simulink model "week8_trial"  (R2020b)
settings: Solver=VariableStepAuto  StartTime=0.0  StopTime=100  FixedStep=0.1  RelTol=1e-3
undefined symbols (not defined in the file or in its folder): Cf, Cr, Iz, lf, lr, m, md, sigbuilder_block, Ts, V_init
libraries: pid_lib x2, mpcadaslib x1
(part 1 of 2)
settings Model: Creator=anime  LastModifiedBy=anime

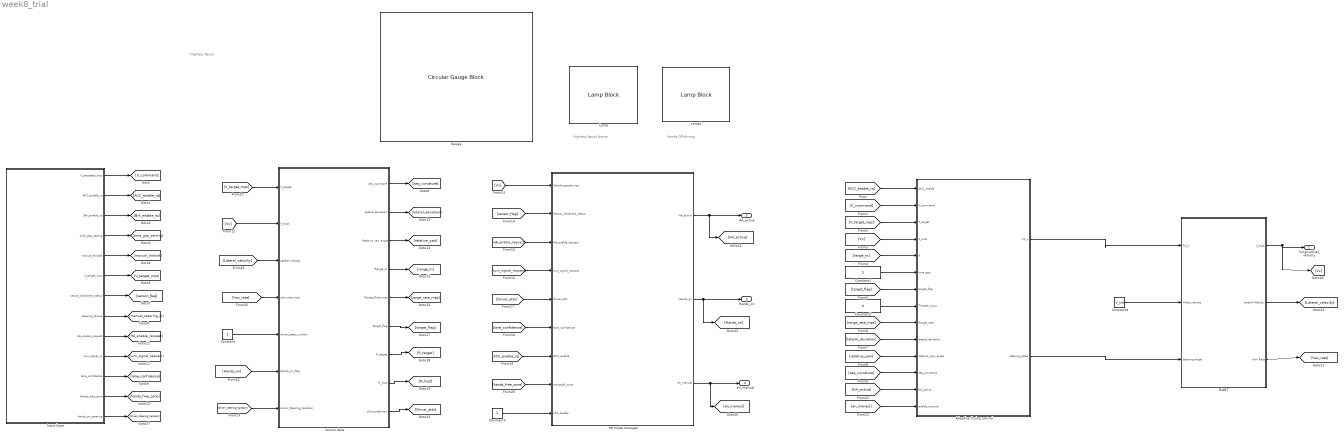
== system week8_trial ==
  note: Hands Off driving
  note: Highway Assist
  note: Highway Assist Active
  Adaptive Cruise control : Subsystem
  Constant : Constant
  Constant1 : Constant  Value=3
  Constant2 : Constant  Value=0
  Constant3 : Constant
  Constant4 : Constant  Value=V_init
  Gauge : CircularGaugeBlock  LabelPosition=Bottom  ScaleMax=50
  HA mode manager : Subsystem
  Input layer : Subsystem
  Lamp : LampBlock  LabelPosition=Bottom
  Lamp1 : LampBlock  LabelPosition=Bottom
  PLANT : Subsystem
  "Sensor data " : Subsystem
  longitudinal_velocity : Outport  Unit=m/s  VectorParamsAs1DForOutWhenUnconnected=off
  HA_active : Outport  Port=2
  Hands_on : Outport  Port=3
  en_manual : Outport  Port=4
  wires:
  Input layer/5(manual_throttle) -> [manual_throttle]
  Input layer/12(Hands_free_zone) -> [hands_free_zone]
  Input layer/11(lane_confidence) -> [lane_confidence]
  Input layer/10(turn_signal_rq) -> [turn_signal_request]
  Input layer/6(V_target_mps) -> [V_target_mps]
  Input layer/9(HA_enable_request) -> [HA_enable_request]
  Input layer/3(Brk_enable_rq) -> [Brk_enable_rq]
  Input layer/8(steering_torque) -> [manual_steering_io]
  Input layer/7(sensor_hardware_status) -> [sensor_flag]
  Input layer/4(time_gap_setting) -> [time_gap_setting]
  Input layer/1(V_setspeed_mps) -> [V_command]
  Input layer/2(ACC_enable_rq) -> [ACC_enable_rq]
  "Sensor data "/9(drive_attention) -> [Driver_attn]
  "Sensor data "/6(Target_flag) -> [target_flag]
  [Yaw_rate] -> "Sensor data "/4(yaw_rate_mps)
  "Sensor data "/8(R_host) -> [R_host]
  "Sensor data "/7(R_target) -> [R_target]
  "Sensor data "/4(Range_m) -> [range_m]
  "Sensor data "/3(Relative yaw angle) -> [relative_yaw]
  [Vx] -> "Sensor data "/2(V_host)
  "Sensor data "/5(Range_Rate_mps) -> [range_rate_mps]
  "Sensor data "/2(Lateral deviation) -> [lateral_deviation]
  [V_target_mps] -> "Sensor data "/1(V_target)
  [Lateral_velocity] -> "Sensor data "/3(Lateral velocity)
  Constant/1 -> "Sensor data "/5(driver_state_monitor)
  "Sensor data "/1(seq_curvature) -> [seq_curvature]
  Constant4/1 -> PLANT/2(initial_velocity)
  [ACC_enable_rq] -> Adaptive Cruise control/1(ACC_enable)
  [V_command] -> Adaptive Cruise control/2(V_command)
  [V_target_mps] -> Adaptive Cruise control/3(V_target)
  [Vx] -> Adaptive Cruise control/4(V_host)
  [range_m] -> Adaptive Cruise control/5(R)
  [target_flag] -> Adaptive Cruise control/7(target_flag)
  Constant1/1 -> Adaptive Cruise control/6(time gap)
  Constant2/1 -> Adaptive Cruise control/8(Throttle_input)
  [range_rate_mps] -> Adaptive Cruise control/9(Range_rate)
  Adaptive Cruise control/1(Fd_u) -> PLANT/1(Fd_U)
  [lateral_deviation] -> Adaptive Cruise control/10(lateral_deviation)
  [relative_yaw] -> Adaptive Cruise control/11(relative_yaw_angle)
  [seq_curvature] -> Adaptive Cruise control/12(seq_curvature)
  HA mode manager/1(HA_active) -> [HA_active], HA_active/1
  HA mode manager/3(en_manual) -> [en_manaul], en_manual/1
  HA mode manager/2(Hands_on) -> [Hands_on], Hands_on/1
  [Vx] -> HA mode manager/1(Vehicle_speed_mps)
  [sensor_flag] -> HA mode manager/2(Sensor_hardware_status)
  [HA_enable_request] -> HA mode manager/3(HA_enable_request)
  [turn_signal_request] -> HA mode manager/4(turn_signal_request)
  [Driver_attn] -> HA mode manager/5(driver_attn)
  [lane_confidence] -> HA mode manager/6(lane_confidence)
  [ACC_enable_rq] -> HA mode manager/7(ACC_enable)
  [hands_free_zone] -> HA mode manager/8(Handsoff_zone)
  Constant3/1 -> HA mode manager/9(LCA_enable)
  [HA_active] -> Adaptive Cruise control/13(HA_active)
  [en_manaul] -> Adaptive Cruise control/14(enable_manual)
  Input layer/13(hands_on_steering) -> [driver_steering_handson]
  [driver_steering_handson] -> "Sensor data "/7(driver_Steering_handson)
  [Hands_on] -> "Sensor data "/6(Hands_on_flag)
  Adaptive Cruise control/2(steering_delta) -> PLANT/3(Steering angle)
  PLANT/1(V_host) -> [Vx], longitudinal_velocity/1
  PLANT/2(Lateral Velocity) -> [Lateral_velocity]
  PLANT/3(Yaw Rate) -> [Yaw_rate]

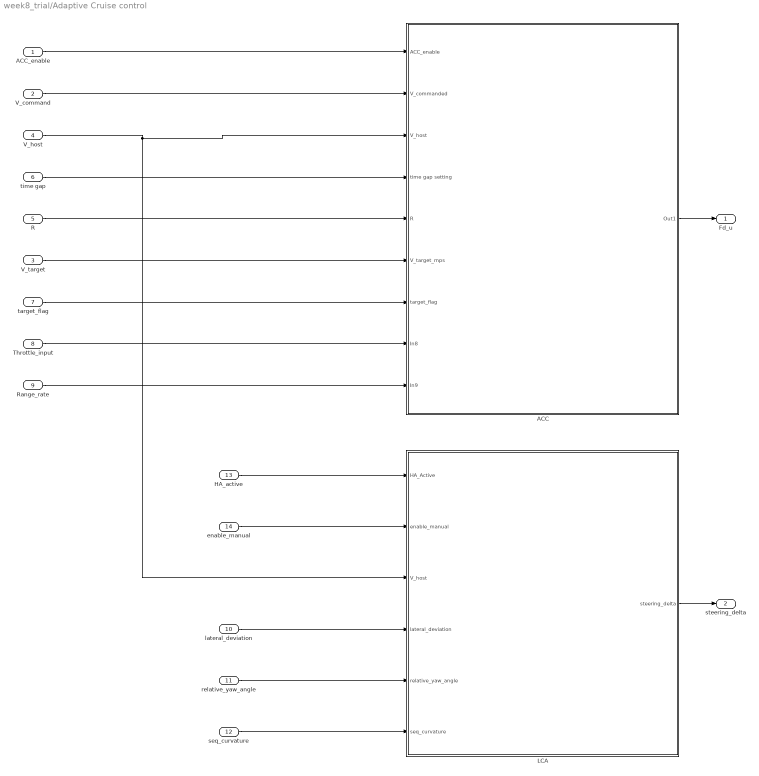
== system week8_trial/Adaptive Cruise control ==
  ACC_enable : Inport
  V_command : Inport  Port=2
  V_target : Inport  Port=3
  V_host : Inport  Port=4
  R : Inport  Port=5
  time gap : Inport  Port=6
  target_flag : Inport  Port=7
  Throttle_input : Inport  Port=8
  Range_rate : Inport  Port=9
  lateral_deviation : Inport  Port=10
  relative_yaw_angle : Inport  Port=11
  seq_curvature : Inport  Port=12
  HA_active : Inport  Port=13
  enable_manual : Inport  Port=14
  ACC : Subsystem
  LCA : Subsystem
  Fd_u : Outport
  steering_delta : Outport  Port=2
  wires:
  ACC_enable/1 -> ACC/1(ACC_enable)
  V_command/1 -> ACC/2(V_commanded)
  V_host/1 -> LCA/3(V_host), ACC/3(V_host)
  time gap/1 -> ACC/4(time gap setting)
  R/1 -> ACC/5(R)
  V_target/1 -> ACC/6(V_target_mps)
  target_flag/1 -> ACC/7(target_flag)
  Throttle_input/1 -> ACC/8(In8)
  Range_rate/1 -> ACC/9(In9)
  ACC/1(Out1) -> Fd_u/1
  HA_active/1 -> LCA/1(HA_Active)
  enable_manual/1 -> LCA/2(enable_manual)
  lateral_deviation/1 -> LCA/4(lateral_deviation)
  relative_yaw_angle/1 -> LCA/5(relative_yaw_angle)
  seq_curvature/1 -> LCA/6(seq_curvature)
  LCA/1(steering_delta) -> steering_delta/1

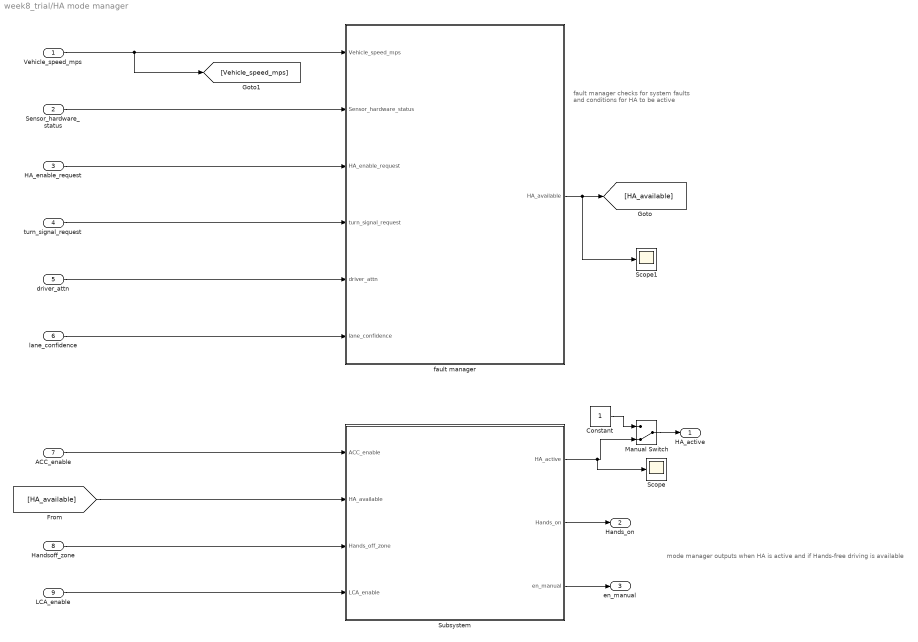
== system week8_trial/HA mode manager ==
  note: mode manager outputs when HA is active and if Hands-free driving is available
  note: fault manager checks for system faults
      | and conditions for HA to be active
  Vehicle_speed_mps : Inport
  Sensor_hardware_status : Inport  Port=2
  HA_enable_request : Inport  Port=3
  turn_signal_request : Inport  Port=4
  driver_attn : Inport  Port=5
  lane_confidence : Inport  Port=6
  ACC_enable : Inport  Port=7
  Handsoff_zone : Inport  Port=8
  LCA_enable : Inport  Port=9
  Constant : Constant
  Manual Switch : ManualSwitch  CurrentSetting=0
  Scope : Scope
  Scope1 : Scope
  Subsystem : Subsystem
  fault manager : Subsystem
  HA_active : Outport
  Hands_on : Outport  Port=2
  en_manual : Outport  Port=3
  wires:
  Vehicle_speed_mps/1 -> [Vehicle_speed_mps], fault manager/1(Vehicle_speed_mps)
  Sensor_hardware_status/1 -> fault manager/2(Sensor_hardware_status)
  HA_enable_request/1 -> fault manager/3(HA_enable_request)
  turn_signal_request/1 -> fault manager/4(turn_signal_request)
  driver_attn/1 -> fault manager/5(driver_attn)
  lane_confidence/1 -> fault manager/6(lane_confidence)
  fault manager/1(HA_available) -> Scope1/1, [HA_available]
  ACC_enable/1 -> Subsystem/1(ACC_enable)
  Handsoff_zone/1 -> Subsystem/3(Hands_off_zone)
  LCA_enable/1 -> Subsystem/4(LCA_enable)
  [HA_available] -> Subsystem/2(HA_available)
  Subsystem/2(Hands_on) -> Hands_on/1
  Subsystem/3(en_manual) -> en_manual/1
  Manual Switch/1 -> HA_active/1
  Constant/1 -> Manual Switch/1
  Subsystem/1(HA_active) -> Scope/1, Manual Switch/2

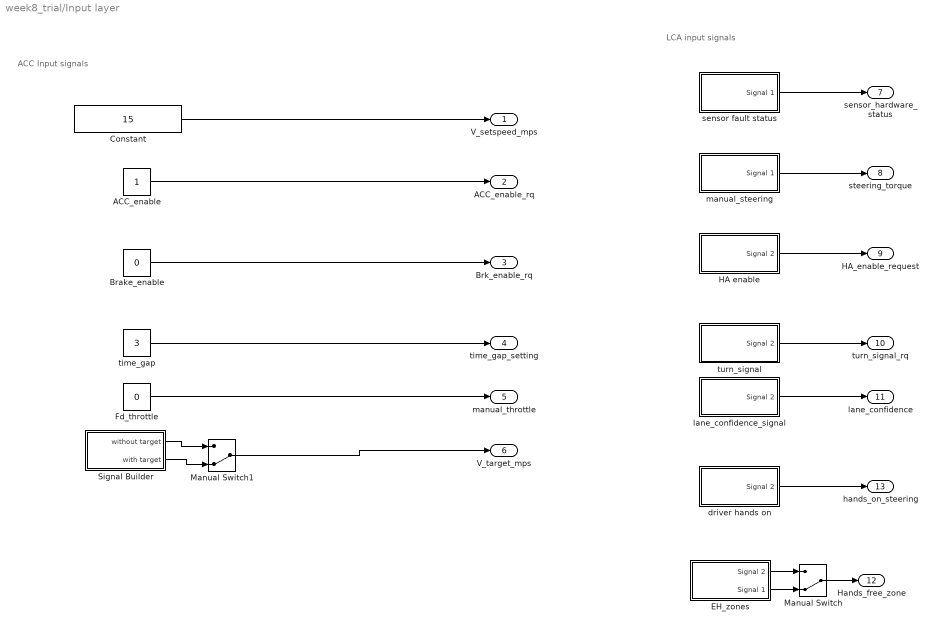
== system week8_trial/Input layer ==
  note: LCA input signals
  note: ACC Input signals
  ACC_enable : Constant
  Brake_enable : Constant  Value=0
  Constant : Constant  Value=15
  EH_zones : Subsystem  Tag=STV Subsys  LoadFcn=sigbuilder_block('load');  StartFcn=sigbuilder_block('start');  StopFcn=sigbuilder_block('stop');  ClipboardFcn=sigbuilder_block('clipboard');  mask(Sigbuilder block){tuvar=[0:10]}
      mask help: Simulink:masks:SigbuilderBlock_MD
      mask init:
      | if ~strcmp(get_param(bdroot(gcbh),'SimulationStatus'),'stopped') tuvar = sigbuilder_block('maskInit'); end
      settings: CopyFcn=sigbuilder_block('copy');  DeleteFcn=sigbuilder_block('delete');  ModelCloseFcn=sigbuilder_block('modelClose');  PreSaveFcn=sigbuilder_block('preSave');  PauseFcn=sigbuilder_block('pause');  ContinueFcn=sigbuilder_block('continue');  NameChangeFcn=sigbuilder_block('namechange');  OpenFcn=sigbuilder_block('open',[883.5 181.5 550.5 359.25 ]);  CloseFcn=sigbuilder_block('close');
      mask Display: plot(0, 0, 100, 100,[2, 2, 32, 32, 2], [68, 8, 8, 68, 68],[32, 2], [38, 38], [32, 19, 2],[53, 60, 44], [32, 17, 17, 2],[16, 16, 31, 31]);txt = getActiveGroup(gcbh);text(2, 100, txt,'verticalAlignment', 'top');
  Fd_throttle : Constant  Value=0  SampleTime=-1
  HA enable : Subsystem  Tag=STV Subsys  LoadFcn=sigbuilder_block('load');  StartFcn=sigbuilder_block('start');  StopFcn=sigbuilder_block('stop');  ClipboardFcn=sigbuilder_block('clipboard');  mask(Sigbuilder block){tuvar=[0:10]}
      mask help: Simulink:masks:SigbuilderBlock_MD
      mask init:
      | if ~strcmp(get_param(bdroot(gcbh),'SimulationStatus'),'stopped') tuvar = sigbuilder_block('maskInit'); end
      settings: CopyFcn=sigbuilder_block('copy');  DeleteFcn=sigbuilder_block('delete');  ModelCloseFcn=sigbuilder_block('modelClose');  PreSaveFcn=sigbuilder_block('preSave');  PauseFcn=sigbuilder_block('pause');  ContinueFcn=sigbuilder_block('continue');  NameChangeFcn=sigbuilder_block('namechange');  OpenFcn=sigbuilder_block('open',[437.6 199.2 550.4 400 ]);  CloseFcn=sigbuilder_block('close');
      mask Display: plot(0, 0, 100, 100,[2, 2, 32, 32, 2], [68, 8, 8, 68, 68],[32, 2], [38, 38], [32, 19, 2],[53, 60, 44], [32, 17, 17, 2],[16, 16, 31, 31]);txt = getActiveGroup(gcbh);text(2, 100, txt,'verticalAlignment', 'top');
  Manual Switch : ManualSwitch  CurrentSetting=0
  Manual Switch1 : ManualSwitch  CurrentSetting=0
  Signal Builder : Subsystem  Tag=STV Subsys  LoadFcn=sigbuilder_block('load',[883.5 164.25 550.5 359.25 ]);  StartFcn=sigbuilder_block('start');  StopFcn=sigbuilder_block('stop');  ClipboardFcn=sigbuilder_block('clipboard');  mask(Sigbuilder block){tuvar=[0:10]}
      mask help: Simulink:masks:SigbuilderBlock_MD
      mask init:
      | if ~strcmp(get_param(bdroot(gcbh),'SimulationStatus'),'stopped') tuvar = sigbuilder_block('maskInit'); end
      settings: CopyFcn=sigbuilder_block('copy');  DeleteFcn=sigbuilder_block('delete');  ModelCloseFcn=sigbuilder_block('modelClose');  PreSaveFcn=sigbuilder_block('preSave');  PauseFcn=sigbuilder_block('pause');  ContinueFcn=sigbuilder_block('continue');  NameChangeFcn=sigbuilder_block('namechange');  OpenFcn=sigbuilder_block('open',[1759.5 164.25 550.5 399.75 ]);  CloseFcn=sigbuilder_block('close');
      mask Display: plot(0, 0, 100, 100,[2, 2, 32, 32, 2], [68, 8, 8, 68, 68],[32, 2], [38, 38], [32, 19, 2],[53, 60, 44], [32, 17, 17, 2],[16, 16, 31, 31]);txt = getActiveGroup(gcbh);text(2, 100, txt,'verticalAlignment', 'top');
  "driver hands on " : Subsystem  Tag=STV Subsys  LoadFcn=sigbuilder_block('load');  StartFcn=sigbuilder_block('start');  StopFcn=sigbuilder_block('stop');  ClipboardFcn=sigbuilder_block('clipboard');  mask(Sigbuilder block){tuvar=[0:10]}
      mask help: Simulink:masks:SigbuilderBlock_MD
      mask init:
      | if ~strcmp(get_param(bdroot(gcbh),'SimulationStatus'),'stopped') tuvar = sigbuilder_block('maskInit'); end
      settings: CopyFcn=sigbuilder_block('copy');  DeleteFcn=sigbuilder_block('delete');  ModelCloseFcn=sigbuilder_block('modelClose');  PreSaveFcn=sigbuilder_block('preSave');  PauseFcn=sigbuilder_block('pause');  ContinueFcn=sigbuilder_block('continue');  NameChangeFcn=sigbuilder_block('namechange');  OpenFcn=sigbuilder_block('open',[437.6 199.2 550.4 400 ]);  CloseFcn=sigbuilder_block('close');
      mask Display: plot(0, 0, 100, 100,[2, 2, 32, 32, 2], [68, 8, 8, 68, 68],[32, 2], [38, 38], [32, 19, 2],[53, 60, 44], [32, 17, 17, 2],[16, 16, 31, 31]);txt = getActiveGroup(gcbh);text(2, 100, txt,'verticalAlignment', 'top');
  lane_confidence_signal : Subsystem  Tag=STV Subsys  LoadFcn=sigbuilder_block('load');  StartFcn=sigbuilder_block('start');  StopFcn=sigbuilder_block('stop');  ClipboardFcn=sigbuilder_block('clipboard');  mask(Sigbuilder block){tuvar=[0:10]}
      mask help: Simulink:masks:SigbuilderBlock_MD
      mask init:
      | if ~strcmp(get_param(bdroot(gcbh),'SimulationStatus'),'stopped') tuvar = sigbuilder_block('maskInit'); end
      settings: CopyFcn=sigbuilder_block('copy');  DeleteFcn=sigbuilder_block('delete');  ModelCloseFcn=sigbuilder_block('modelClose');  PreSaveFcn=sigbuilder_block('preSave');  PauseFcn=sigbuilder_block('pause');  ContinueFcn=sigbuilder_block('continue');  NameChangeFcn=sigbuilder_block('namechange');  OpenFcn=sigbuilder_block('open',[437.6 199.2 550.4 400 ]);  CloseFcn=sigbuilder_block('close');
      mask Display: plot(0, 0, 100, 100,[2, 2, 32, 32, 2], [68, 8, 8, 68, 68],[32, 2], [38, 38], [32, 19, 2],[53, 60, 44], [32, 17, 17, 2],[16, 16, 31, 31]);txt = getActiveGroup(gcbh);text(2, 100, txt,'verticalAlignment', 'top');
  manual_steering : Subsystem  Tag=STV Subsys  LoadFcn=sigbuilder_block('load');  StartFcn=sigbuilder_block('start');  StopFcn=sigbuilder_block('stop');  ClipboardFcn=sigbuilder_block('clipboard');  mask(Sigbuilder block){tuvar=[0:10]}
      mask help: Simulink:masks:SigbuilderBlock_MD
      mask init:
      | if ~strcmp(get_param(bdroot(gcbh),'SimulationStatus'),'stopped') tuvar = sigbuilder_block('maskInit'); end
      settings: CopyFcn=sigbuilder_block('copy');  DeleteFcn=sigbuilder_block('delete');  ModelCloseFcn=sigbuilder_block('modelClose');  PreSaveFcn=sigbuilder_block('preSave');  PauseFcn=sigbuilder_block('pause');  ContinueFcn=sigbuilder_block('continue');  NameChangeFcn=sigbuilder_block('namechange');  OpenFcn=sigbuilder_block('open',[437.6 199.2 550.4 400 ]);  CloseFcn=sigbuilder_block('close');
      mask Display: plot(0, 0, 100, 100,[2, 2, 32, 32, 2], [68, 8, 8, 68, 68],[32, 2], [38, 38], [32, 19, 2],[53, 60, 44], [32, 17, 17, 2],[16, 16, 31, 31]);txt = getActiveGroup(gcbh);text(2, 100, txt,'verticalAlignment', 'top');
  sensor fault status : Subsystem  Tag=STV Subsys  LoadFcn=sigbuilder_block('load');  StartFcn=sigbuilder_block('start');  StopFcn=sigbuilder_block('stop');  ClipboardFcn=sigbuilder_block('clipboard');  mask(Sigbuilder block){tuvar=[0:10]}
      mask help: Simulink:masks:SigbuilderBlock_MD
      mask init:
      | if ~strcmp(get_param(bdroot(gcbh),'SimulationStatus'),'stopped') tuvar = sigbuilder_block('maskInit'); end
      settings: CopyFcn=sigbuilder_block('copy');  DeleteFcn=sigbuilder_block('delete');  ModelCloseFcn=sigbuilder_block('modelClose');  PreSaveFcn=sigbuilder_block('preSave');  PauseFcn=sigbuilder_block('pause');  ContinueFcn=sigbuilder_block('continue');  NameChangeFcn=sigbuilder_block('namechange');  OpenFcn=sigbuilder_block('open',[437.6 199.2 550.4 400 ]);  CloseFcn=sigbuilder_block('close');
      mask Display: plot(0, 0, 100, 100,[2, 2, 32, 32, 2], [68, 8, 8, 68, 68],[32, 2], [38, 38], [32, 19, 2],[53, 60, 44], [32, 17, 17, 2],[16, 16, 31, 31]);txt = getActiveGroup(gcbh);text(2, 100, txt,'verticalAlignment', 'top');
  time_gap : Constant  Value=3
  turn_signal : Subsystem  Tag=STV Subsys  LoadFcn=sigbuilder_block('load');  StartFcn=sigbuilder_block('start');  StopFcn=sigbuilder_block('stop');  ClipboardFcn=sigbuilder_block('clipboard');  mask(Sigbuilder block){tuvar=[0:10]}
      mask help: Simulink:masks:SigbuilderBlock_MD
      mask init:
      | if ~strcmp(get_param(bdroot(gcbh),'SimulationStatus'),'stopped') tuvar = sigbuilder_block('maskInit'); end
      settings: CopyFcn=sigbuilder_block('copy');  DeleteFcn=sigbuilder_block('delete');  ModelCloseFcn=sigbuilder_block('modelClose');  PreSaveFcn=sigbuilder_block('preSave');  PauseFcn=sigbuilder_block('pause');  ContinueFcn=sigbuilder_block('continue');  NameChangeFcn=sigbuilder_block('namechange');  OpenFcn=sigbuilder_block('open',[437.6 199.2 550.4 400 ]);  CloseFcn=sigbuilder_block('close');
      mask Display: plot(0, 0, 100, 100,[2, 2, 32, 32, 2], [68, 8, 8, 68, 68],[32, 2], [38, 38], [32, 19, 2],[53, 60, 44], [32, 17, 17, 2],[16, 16, 31, 31]);txt = getActiveGroup(gcbh);text(2, 100, txt,'verticalAlignment', 'top');
  V_setspeed_mps : Outport
  ACC_enable_rq : Outport  Port=2
  Brk_enable_rq : Outport  Port=3
  time_gap_setting : Outport  Port=4
  manual_throttle : Outport  Port=5
  V_target_mps : Outport  Port=6
  sensor_hardware_status : Outport  Port=7
  steering_torque : Outport  Port=8
  HA_enable_request : Outport  Port=9
  turn_signal_rq : Outport  Port=10
  lane_confidence : Outport  Port=11
  Hands_free_zone : Outport  Port=12
  hands_on_steering : Outport  Port=13
  wires:
  Constant/1 -> V_setspeed_mps/1
  ACC_enable/1 -> ACC_enable_rq/1
  Brake_enable/1 -> Brk_enable_rq/1
  time_gap/1 -> time_gap_setting/1
  Fd_throttle/1 -> manual_throttle/1
  sensor fault status/1(Signal 1) -> sensor_hardware_status/1
  manual_steering/1(Signal 1) -> steering_torque/1
  HA enable/1(Signal 2) -> HA_enable_request/1
  turn_signal/1(Signal 2) -> turn_signal_rq/1
  lane_confidence_signal/1(Signal 2) -> lane_confidence/1
  "driver hands on "/1(Signal 2) -> hands_on_steering/1
  EH_zones/1(Signal 2) -> Manual Switch/1
  EH_zones/2(Signal 1) -> Manual Switch/2
  Manual Switch/1 -> Hands_free_zone/1
  Signal Builder/1(without target) -> Manual Switch1/1
  Signal Builder/2(with target) -> Manual Switch1/2
  Manual Switch1/1 -> V_target_mps/1

== system week8_trial/PLANT ==
  Fd_U : Inport
  initial_velocity : Inport  Port=2
  Steering angle : Inport  Port=3
  Lateral Vehicle Dynamics : Subsystem
  Longitudinal plant : Subsystem
  Scope : Scope
  V_host : Outport
  Lateral Velocity : Outport  Port=2
  Yaw Rate : Outport  Port=3
  wires:
  Fd_U/1 -> Longitudinal plant/1(Fd_U)
  initial_velocity/1 -> Longitudinal plant/2(initial_velocity)
  Longitudinal plant/1(V_host) -> Lateral Vehicle Dynamics/1(Longitudinal velocity), Scope/1, V_host/1  "V_host"
  Lateral Vehicle Dynamics/1(Lateral Velocity) -> Lateral Velocity/1
  Lateral Vehicle Dynamics/2(Yaw Rate) -> Yaw Rate/1
  Steering angle/1 -> Lateral Vehicle Dynamics/2(Steering angle)

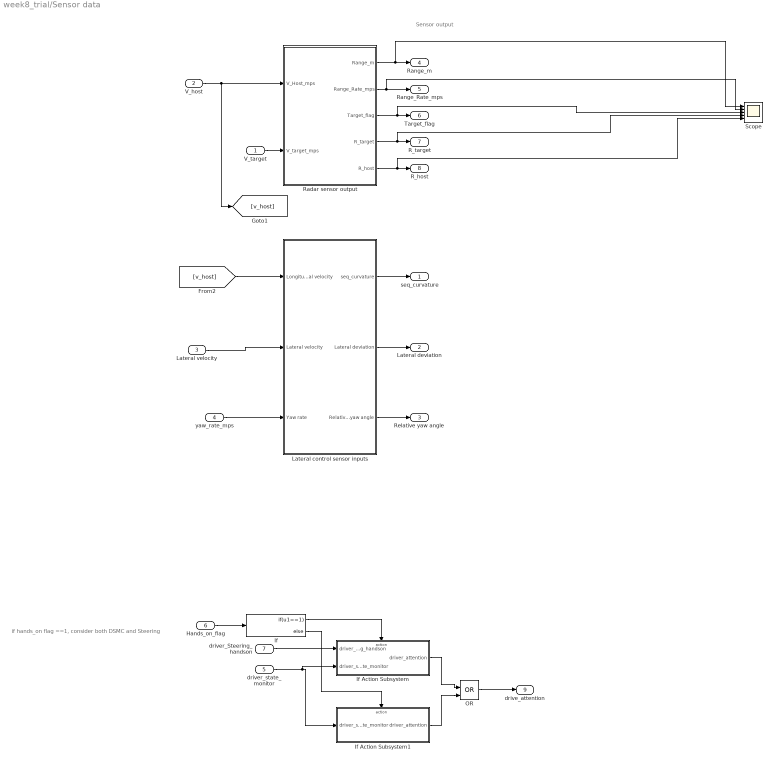
== system week8_trial/Sensor data  ==
  note: if hands_on flag ==1, consider both DSMC and Steering
  note: Sensor output
  V_target : Inport
  V_host : Inport  Port=2
  Lateral velocity : Inport  Port=3
  yaw_rate_mps : Inport  Port=4
  driver_state_monitor : Inport  Port=5
  Hands_on_flag : Inport  Port=6
  driver_Steering_handson : Inport  Port=7
  If : If  IfExpression=u1==1
  If Action Subsystem : Subsystem  TreatAsAtomicUnit=on
  If Action Subsystem1 : Subsystem  TreatAsAtomicUnit=on
  Lateral control sensor inputs : Subsystem
  OR : Logic  Operator=OR  IconShape=distinctive  AllPortsSameDT=off  OutDataTypeStr=boolean
  Radar sensor output : Subsystem
  Scope : Scope  NumInputPorts=5
  seq_curvature : Outport
  Lateral deviation : Outport  Port=2
  Relative yaw angle : Outport  Port=3
  Range_m : Outport  Port=4
  Range_Rate_mps : Outport  Port=5
  Target_flag : Outport  Port=6
  R_target : Outport  Port=7
  R_host : Outport  Port=8
  drive_attention : Outport  Port=9
  wires:
  V_target/1 -> Radar sensor output/2(V_target_mps)
  V_host/1 -> [v_host], Radar sensor output/1(V_Host_mps)
  [v_host] -> Lateral control sensor inputs/1(Longitudinal velocity)
  Lateral velocity/1 -> Lateral control sensor inputs/2(Lateral velocity)
  yaw_rate_mps/1 -> Lateral control sensor inputs/3(Yaw rate)
  Lateral control sensor inputs/1(seq_curvature) -> seq_curvature/1
  Lateral control sensor inputs/2(Lateral deviation) -> Lateral deviation/1
  Lateral control sensor inputs/3(Relative yaw angle) -> Relative yaw angle/1
  Radar sensor output/1(Range_m) -> Scope/1, Range_m/1
  Radar sensor output/2(Range_Rate_mps) -> Scope/2, Range_Rate_mps/1
  Radar sensor output/3(Target_flag) -> Scope/3, Target_flag/1
  Radar sensor output/4(R_target) -> Scope/4, R_target/1
  Radar sensor output/5(R_host) -> Scope/5, R_host/1
  Hands_on_flag/1 -> If/1
  If/1 -> If Action Subsystem/Action
  driver_Steering_handson/1 -> If Action Subsystem/1(driver_Steering_handson)
  driver_state_monitor/1 -> If Action Subsystem1/1(driver_state_monitor), If Action Subsystem/2(driver_state_monitor)
  If/2 -> If Action Subsystem1/Action
  If Action Subsystem/1(driver_attention) -> OR/1
  If Action Subsystem1/1(driver_attention) -> OR/2
  OR/1 -> drive_attention/1

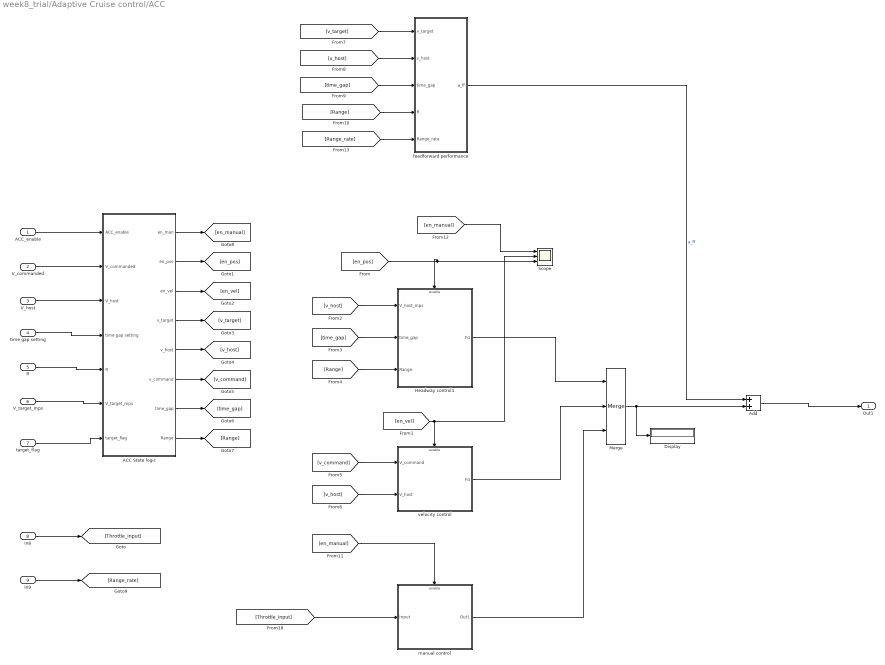
== system week8_trial/Adaptive Cruise control/ACC ==
  ACC_enable : Inport
  V_commanded : Inport  Port=2
  V_host : Inport  Port=3
  time gap setting : Inport  Port=4
  R : Inport  Port=5
  V_target_mps : Inport  Port=6
  target_flag : Inport  Port=7
  In8 : Inport  Port=8
  In9 : Inport  Port=9
  ACC State logic : Subsystem
  Add : Sum
  Display : Display
  Headway control1 : Subsystem
  Merge : Merge  Inputs=3
  Scope : Scope  NumInputPorts=3
  feedforward performance : Subsystem
  manual control : Subsystem
  velocity control : Subsystem
  Out1 : Outport
  wires:
  ACC State logic/1(en_man) -> [en_manual]
  [en_manual] -> Scope/1
  [en_vel] -> velocity control/Enable, Scope/2
  [time_gap] -> Headway control1/2(time_gap)
  [en_pos] -> Headway control1/Enable, Scope/3
  [v_command] -> velocity control/1(V_command)
  [Range] -> feedforward performance/4(R)
  Merge/1 -> Add/2, Display/1
  ACC State logic/2(en_pos) -> [en_pos]
  In9/1 -> [Range_rate]
  [v_host] -> velocity control/2(V_host)
  target_flag/1 -> ACC State logic/7(target_flag)
  V_target_mps/1 -> ACC State logic/6(V_target_mps)
  manual control/1(Out1) -> Merge/3
  ACC State logic/6(v_command) -> [v_command]
  ACC State logic/5(v_host) -> [v_host]
  [Throttle_input] -> manual control/1(Input)
  V_host/1 -> ACC State logic/3(V_host)
  ACC State logic/8(Range) -> [Range]
  ACC State logic/4(v_target) -> [v_target]
  R/1 -> ACC State logic/5(R)
  velocity control/1(Fd) -> Merge/2
  time gap setting/1 -> ACC State logic/4(time gap setting)
  [Range] -> Headway control1/3(Range)
  ACC State logic/7(time_gap) -> [time_gap]
  [v_host] -> feedforward performance/2(v_host)
  [v_target] -> feedforward performance/1(v_target)
  [v_host] -> Headway control1/1(V_host_mps)
  ACC_enable/1 -> ACC State logic/1(ACC_enable)
  [Range_rate] -> feedforward performance/5(Range_rate)
  ACC State logic/3(en_vel) -> [en_vel]
  [en_manual] -> manual control/Enable
  [time_gap] -> feedforward performance/3(time_gap)
  Headway control1/1(Fd) -> Merge/1
  feedforward performance/1(a_ff) -> Add/1  "a_ff"
  Add/1 -> Out1/1
  V_commanded/1 -> ACC State logic/2(V_commanded)
  In8/1 -> [Throttle_input]

== system week8_trial/Adaptive Cruise control/LCA ==
  HA_Active : Inport
  enable_manual : Inport  Port=2
  V_host : Inport  Port=3
  lateral_deviation : Inport  Port=4
  relative_yaw_angle : Inport  Port=5
  seq_curvature : Inport  Port=6
  MPC : Subsystem
  Merge : Merge
  manual : Subsystem
  steering_delta : Outport
  wires:
  Merge/1 -> steering_delta/1
  V_host/1 -> MPC/2(V_host_mps)
  lateral_deviation/1 -> MPC/3(lateral_deviation)
  HA_Active/1 -> MPC/Enable
  relative_yaw_angle/1 -> MPC/4(relative_yaw_angle)
  seq_curvature/1 -> MPC/1(seq_curvature)
  enable_manual/1 -> manual/Enable
  manual/1(delta) -> Merge/2
  MPC/1(steering angle (rad)) -> Merge/1

== system week8_trial/HA mode manager/Subsystem ==
  ACC_enable : Inport
  HA_available : Inport  Port=2
  Hands_off_zone : Inport  Port=3
  LCA_enable : Inport  Port=4
  Chart : Stateflow chart  TreatAsAtomicUnit=on
  HA_active : Outport
  Hands_on : Outport  Port=2
  en_manual : Outport  Port=3
  wires:
  ACC_enable/1 -> Chart/1(ACC_enable)
  HA_available/1 -> Chart/2(HA_available)
  Hands_off_zone/1 -> Chart/4(Hands_off_zone)
  LCA_enable/1 -> Chart/3(LCA_enable)
  Chart/1(HA_active) -> HA_active/1
  Chart/2(Hands_on) -> Hands_on/1
  Chart/3(en_manual) -> en_manual/1

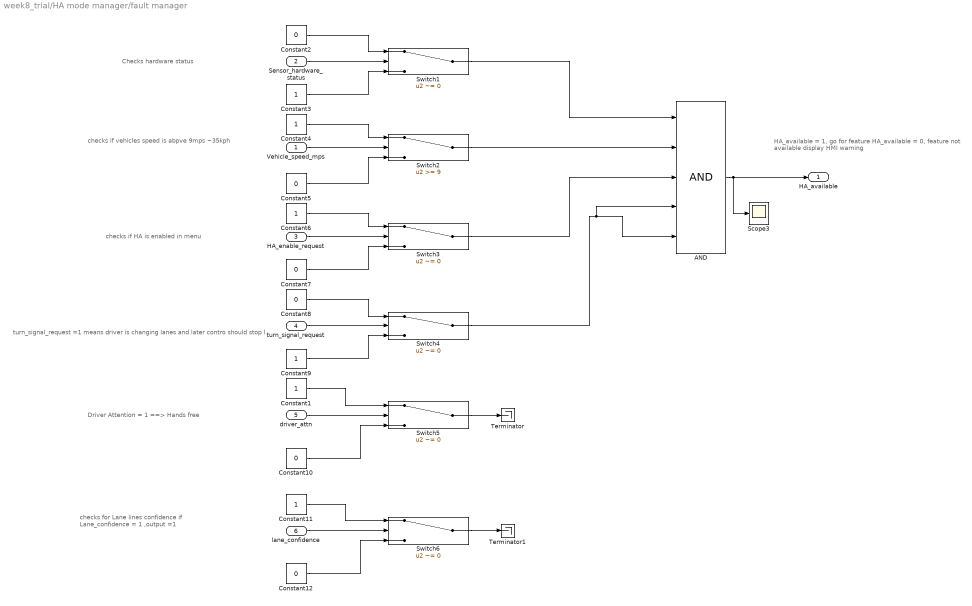
== system week8_trial/HA mode manager/fault manager ==
  note: checks for Lane lines confidence
      | if Lane_confidence = 1 ,output =1
  note: HA_available = 1, go for feature
      | HA_available = 0, feature not available display HMI warning
  note: Driver Attention = 1 ==> Hands free
  note: turn_signal_request =1 means driver is changing lanes and later contro should stop
      | l
  note: checks if HA is enabled in menu
  note: checks if vehicles speed is abpve 9mps ~35kph
  note: Checks hardware status
  Vehicle_speed_mps : Inport
  Sensor_hardware_status : Inport  Port=2
  HA_enable_request : Inport  Port=3
  turn_signal_request : Inport  Port=4
  driver_attn : Inport  Port=5
  lane_confidence : Inport  Port=6
  AND : Logic  Inputs=5  AllPortsSameDT=off  OutDataTypeStr=boolean
  Constant{1,3..4,6,9,11} (6 alike) : Constant
  Constant{2,5,7..8,10,12} (6 alike) : Constant  Value=0
  Scope3 : Scope
  Switch1 : Switch  Criteria=u2 ~= 0
  Switch2 : Switch  Threshold=9
  Switch{3..6} (4 alike) : Switch  Criteria=u2 ~= 0  Threshold=10
  Terminator : Terminator
  Terminator1 : Terminator
  HA_available : Outport
  wires:
  Switch1/1 -> AND/1
  Constant9/1 -> Switch4/3
  Switch4/1 -> AND/4, AND/5
  Constant8/1 -> Switch4/1
  turn_signal_request/1 -> Switch4/2
  Switch3/1 -> AND/3
  Switch2/1 -> AND/2
  Constant7/1 -> Switch3/3
  Constant6/1 -> Switch3/1
  HA_enable_request/1 -> Switch3/2
  Constant3/1 -> Switch1/3
  Constant2/1 -> Switch1/1
  Constant4/1 -> Switch2/1
  Constant5/1 -> Switch2/3
  Sensor_hardware_status/1 -> Switch1/2
  Vehicle_speed_mps/1 -> Switch2/2
  AND/1 -> Scope3/1, HA_available/1
  driver_attn/1 -> Switch5/2
  Constant1/1 -> Switch5/1
  Constant10/1 -> Switch5/3
  Switch5/1 -> Terminator/1
  Constant12/1 -> Switch6/3
  Switch6/1 -> Terminator1/1
  lane_confidence/1 -> Switch6/2
  Constant11/1 -> Switch6/1

== system week8_trial/Input layer/EH_zones ==
  Demux : Demux  Tag=STV Demux  Outputs=2
      settings: DisplayOption=none
  FromWs : FromWorkspace  Tag=STV FromWs  VariableName=tuvar
      SigBuilderData=|
      | common.afterFinalStr = 'Extrapolate'
      | common.sampleTime = 0
      | dataSet.timeRange = [0 16]
      | dataSet.name = 'Group 1'
      | sbobj.Groups.Name = 'Group 1'
      | sbobj.Groups.Signals(1).Name = 'Signal 2'
      | sbobj.Groups.Signals(1).XData = [0 16]
      | sbobj.Groups.Signals(1).YData = [1 1]
      | sbobj.Groups.Signals(2).Name = 'Signal 1'
      | sbobj.Groups.Signals(2).XData = [0 8 8 16]
      | sbobj.Groups.Signals(2).YData = [0 0 1 1]
      | sbobj.Groups.TimeRange = [0 16]
  Signal 2 : Outport  Tag=STV Outport
  Signal 1 : Outport  Tag=STV Outport  Port=2
  wires:
  Demux/1 -> Signal 2/1
  FromWs/1 -> Demux/1
  Demux/2 -> Signal 1/1

== system week8_trial/Input layer/HA enable ==
  Demux : Demux  Tag=STV Demux  Outputs=1
      settings: DisplayOption=none
  FromWs : FromWorkspace  Tag=STV FromWs  VariableName=tuvar
      SigBuilderData=|
      | common.afterFinalStr = 'Extrapolate'
      | common.sampleTime = 0
      | dataSet.timeRange = [0 10]
      | dataSet.name = 'Group 1'
      | sbobj.Groups.Name = 'Group 1'
      | sbobj.Groups.Signals.Name = 'Signal 2'
      | sbobj.Groups.Signals.XData = [0 10]
      | sbobj.Groups.Signals.YData = [1 1]
  Signal 2 : Outport  Tag=STV Outport
  wires:
  FromWs/1 -> Demux/1
  Demux/1 -> Signal 2/1

== system week8_trial/Input layer/Signal Builder ==
  Demux : Demux  Tag=STV Demux  Outputs=2
      settings: DisplayOption=none
  FromWs : FromWorkspace  Tag=STV FromWs  VariableName=tuvar
      SigBuilderData=|
      | common.afterFinalStr = 'Extrapolate'
      | common.sampleTime = 0
      | dataSet.timeRange = [0 100]
      | dataSet.name = 'Group 1'
      | sbobj.Groups.Name = 'Group 1'
      | sbobj.Groups.Signals(1).Name = 'without target'
      | sbobj.Groups.Signals(1).XData = [0 100]
      | sbobj.Groups.Signals(1).YData = [0 0]
      | sbobj.Groups.Signals(2).Name = 'with target'
      | sbobj.Groups.Signals(2).XData = [0 8.5 8.5 100]
      | sbobj.Groups.Signals(2).YData = [27 27 10 10]
      | sbobj.Groups.TimeRange = [0 100]
  without target : Outport  Tag=STV Outport
  with target : Outport  Tag=STV Outport  Port=2
  wires:
  FromWs/1 -> Demux/1
  Demux/1 -> without target/1
  Demux/2 -> with target/1

== system week8_trial/Input layer/driver hands on  ==
  Demux : Demux  Tag=STV Demux  Outputs=1
      settings: DisplayOption=none
  FromWs : FromWorkspace  Tag=STV FromWs  VariableName=tuvar
      SigBuilderData=|
      | common.afterFinalStr = 'Extrapolate'
      | common.sampleTime = 0
      | dataSet.timeRange = [0 10]
      | dataSet.name = 'Group 1'
      | sbobj.Groups.Name = 'Group 1'
      | sbobj.Groups.Signals.Name = 'Signal 2'
      | sbobj.Groups.Signals.XData = [0 10]
      | sbobj.Groups.Signals.YData = [1 1]
  Signal 2 : Outport  Tag=STV Outport
  wires:
  Demux/1 -> Signal 2/1
  FromWs/1 -> Demux/1

== system week8_trial/Input layer/lane_confidence_signal ==
  Demux : Demux  Tag=STV Demux  Outputs=1
      settings: DisplayOption=none
  FromWs : FromWorkspace  Tag=STV FromWs  VariableName=tuvar
      SigBuilderData=|
      | common.afterFinalStr = 'Extrapolate'
      | common.sampleTime = 0
      | dataSet.timeRange = [0 10]
      | dataSet.name = 'Group 1'
      | sbobj.Groups.Name = 'Group 1'
      | sbobj.Groups.Signals.Name = 'Signal 2'
      | sbobj.Groups.Signals.XData = [0 10]
      | sbobj.Groups.Signals.YData = [1 1]
  Signal 2 : Outport  Tag=STV Outport
  wires:
  FromWs/1 -> Demux/1
  Demux/1 -> Signal 2/1

== system week8_trial/Input layer/manual_steering ==
  Demux : Demux  Tag=STV Demux  Outputs=1
      settings: DisplayOption=none
  FromWs : FromWorkspace  Tag=STV FromWs  VariableName=tuvar
      SigBuilderData=|
      | common.afterFinalStr = 'Extrapolate'
      | common.sampleTime = 0
      | dataSet.timeRange = [0 10]
      | dataSet.name = 'Group 1'
      | sbobj.Groups.Name = 'Group 1'
      | sbobj.Groups.Signals.Name = 'Signal 1'
      | sbobj.Groups.Signals.XData = [0 4 6 10]
      | sbobj.Groups.Signals.YData = [0 0 0 0]
  Signal 1 : Outport  Tag=STV Outport
  wires:
  FromWs/1 -> Demux/1
  Demux/1 -> Signal 1/1

== system week8_trial/Input layer/sensor fault status ==
  Demux : Demux  Tag=STV Demux  Outputs=1
      settings: DisplayOption=none
  FromWs : FromWorkspace  Tag=STV FromWs  VariableName=tuvar
      SigBuilderData=|
      | common.afterFinalStr = 'Extrapolate'
      | common.sampleTime = 0
      | dataSet.timeRange = [0 10]
      | dataSet.name = 'Group 1'
      | sbobj.Groups.Name = 'Group 1'
      | sbobj.Groups.Signals.Name = 'Signal 1'
      | sbobj.Groups.Signals.XData = [0 4 6 10]
      | sbobj.Groups.Signals.YData = [0 0 0 0]
  Signal 1 : Outport  Tag=STV Outport
  wires:
  Demux/1 -> Signal 1/1
  FromWs/1 -> Demux/1

== system week8_trial/Input layer/turn_signal ==
  Demux : Demux  Tag=STV Demux  Outputs=1
      settings: DisplayOption=none
  FromWs : FromWorkspace  Tag=STV FromWs  VariableName=tuvar
      SigBuilderData=|
      | common.afterFinalStr = 'Extrapolate'
      | common.sampleTime = 0
      | dataSet.timeRange = [0 10]
      | dataSet.name = 'Group 1'
      | sbobj.Groups.Name = 'Group 1'
      | sbobj.Groups.Signals.Name = 'Signal 2'
      | sbobj.Groups.Signals.XData = [0 10]
      | sbobj.Groups.Signals.YData = [0 0]
  Signal 2 : Outport  Tag=STV Outport
  wires:
  Demux/1 -> Signal 2/1
  FromWs/1 -> Demux/1

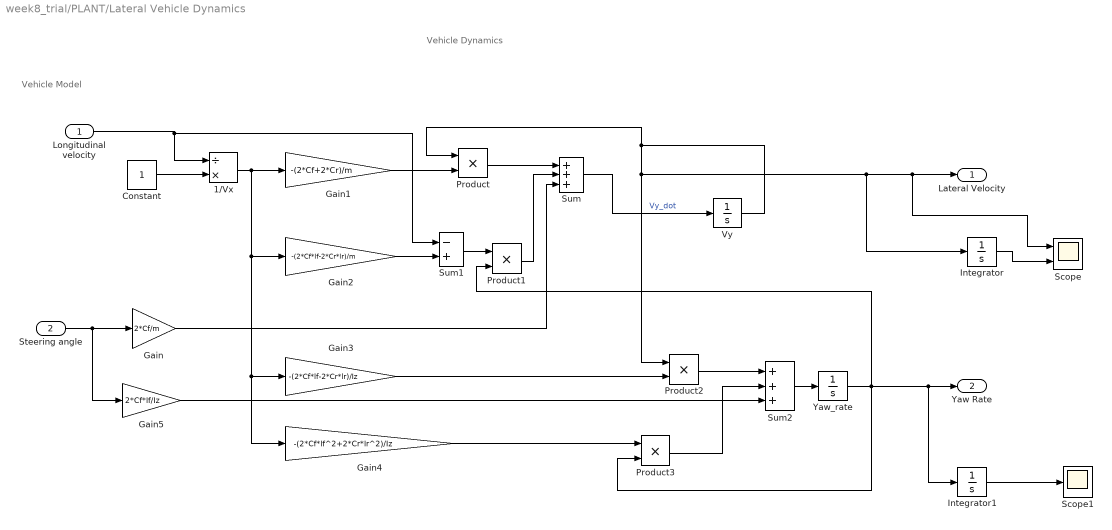
== system week8_trial/PLANT/Lateral Vehicle Dynamics ==
  note: Vehicle Model
  note: Vehicle Dynamics
  Longitudinal velocity : Inport
  Steering angle : Inport  Port=2
  1/Vx : Product  Inputs=/*
  Constant : Constant
  Gain : Gain  Gain=2*Cf/m
  Gain1 : Gain  Gain=-(2*Cf+2*Cr)/m
  Gain2 : Gain  Gain=-(2*Cf*lf-2*Cr*lr)/m
  Gain3 : Gain  Gain=-(2*Cf*lf-2*Cr*lr)/Iz
  Gain4 : Gain  Gain=-(2*Cf*lf^2+2*Cr*lr^2)/Iz
  Gain5 : Gain  Gain=2*Cf*lf/Iz
  Integrator : Integrator
  Integrator1 : Integrator
  Product{,1..3} (4 alike) : Product
  Scope : Scope  NumInputPorts=2
  Scope1 : Scope
  Sum : Sum  Inputs=+++
  Sum1 : Sum  Inputs=-+
  Sum2 : Sum  Inputs=+++
  Vy : Integrator
  "Yaw_rate " : Integrator
  Lateral Velocity : Outport  VectorParamsAs1DForOutWhenUnconnected=off
  Yaw Rate : Outport  Port=2  VectorParamsAs1DForOutWhenUnconnected=off
  wires:
  Integrator1/1 -> Scope1/1
  Sum2/1 -> "Yaw_rate "/1
  Integrator/1 -> Scope/2
  Product1/1 -> Sum/2
  Longitudinal velocity/1 -> Sum1/1, 1/Vx/1
  Product/1 -> Sum/1
  Steering angle/1 -> Gain/1, Gain5/1
  1/Vx/1 -> Gain4/1, Gain3/1, Gain2/1, Gain1/1
  Sum/1 -> Vy/1  "Vy_dot"
  "Yaw_rate "/1 -> Product3/2, Integrator1/1, Yaw Rate/1, Product1/2
  Vy/1 -> Product/1, Integrator/1, Scope/1, Lateral Velocity/1, Product2/1
  Gain/1 -> Sum/3
  Product2/1 -> Sum2/1
  Gain1/1 -> Product/2
  Constant/1 -> 1/Vx/2
  Gain5/1 -> Sum2/3
  Gain3/1 -> Product2/2
  Product3/1 -> Sum2/2
  Gain2/1 -> Sum1/2
  Sum1/1 -> Product1/1
  Gain4/1 -> Product3/1

== system week8_trial/PLANT/Longitudinal plant ==
  Fd_U : Inport
  initial_velocity : Inport  Port=2
  Gain : Gain  Gain=9.211*1e-4
  Gain1 : Gain  Gain=0.0216
  Integrator1 : Integrator  InitialConditionSource=external  InitialCondition=20
  Sum2 : Sum  Inputs=|+-
  V_host : Outport  VectorParamsAs1DForOutWhenUnconnected=off
  wires:
  Gain1/1 -> Sum2/2
  Integrator1/1 -> V_host/1, Gain1/1
  Gain/1 -> Sum2/1
  Fd_U/1 -> Gain/1
  initial_velocity/1 -> Integrator1/2
  Sum2/1 -> Integrator1/1

== system week8_trial/Sensor data /If Action Subsystem ==
  note: driver_attn =1 , good for HA
  driver_Steering_handson : Inport
  driver_state_monitor : Inport  Port=2
  Action Port : ActionPort  ActionPortLabel=if(u1==1)
  AND : Logic  IconShape=distinctive  AllPortsSameDT=off  OutDataTypeStr=boolean
  driver_attention : Outport
  wires:
  driver_Steering_handson/1 -> AND/1
  driver_state_monitor/1 -> AND/2
  AND/1 -> driver_attention/1

== system week8_trial/Sensor data /If Action Subsystem1 ==
  note: driver_attn =1 , good for HA
  driver_state_monitor : Inport
  Action Port : ActionPort  ActionPortLabel=else
  driver_attention : Outport
  wires:
  driver_state_monitor/1 -> driver_attention/1

== system week8_trial/Sensor data /Lateral control sensor inputs ==
  note: LATERAL DYNAMICS FOR MPC
  Longitudinal velocity : Inport
  Lateral velocity : Inport  Port=2
  Yaw rate : Inport  Port=3
  Sensor Dynamics : Subsystem
  Subsystem : Subsystem  mask{signal=md, ts=Ts, steps=10}
      mask prompts: signal "Signal name"; ts "Sampling time"; steps "Number of previewing steps"
      mask init:
      | ts = evalin('base',get_param(gcbh,'ts'));
      | signal = evalin('base',get_param(gcbh,'signal'));
      | steps = evalin('base',get_param(gcbh,'steps'));
      | data = mpc_previewer_maskinit(signal,ts);
      mask Display:
      | fprintf('Future\nsample\nextractor');
      | port_label('output', 1, 'seq')
      | port_label('output', 2, '@t')
  seq_curvature : Outport
  Lateral deviation : Outport  Port=2
  Relative yaw angle : Outport  Port=3
  wires:
  Subsystem/2(current) -> Sensor Dynamics/1(Current curvature)
  Subsystem/1(sequence) -> seq_curvature/1
  Longitudinal velocity/1 -> Sensor Dynamics/2(Longitudinal velocity)
  Lateral velocity/1 -> Sensor Dynamics/3(Lateral velocity)
  Yaw rate/1 -> Sensor Dynamics/4(Yaw rate)
  Sensor Dynamics/1(Lateral deviation) -> Lateral deviation/1  "lateral_deviation"
  Sensor Dynamics/2(Relative yaw angle) -> Relative yaw angle/1  "relative_yaw_angle"

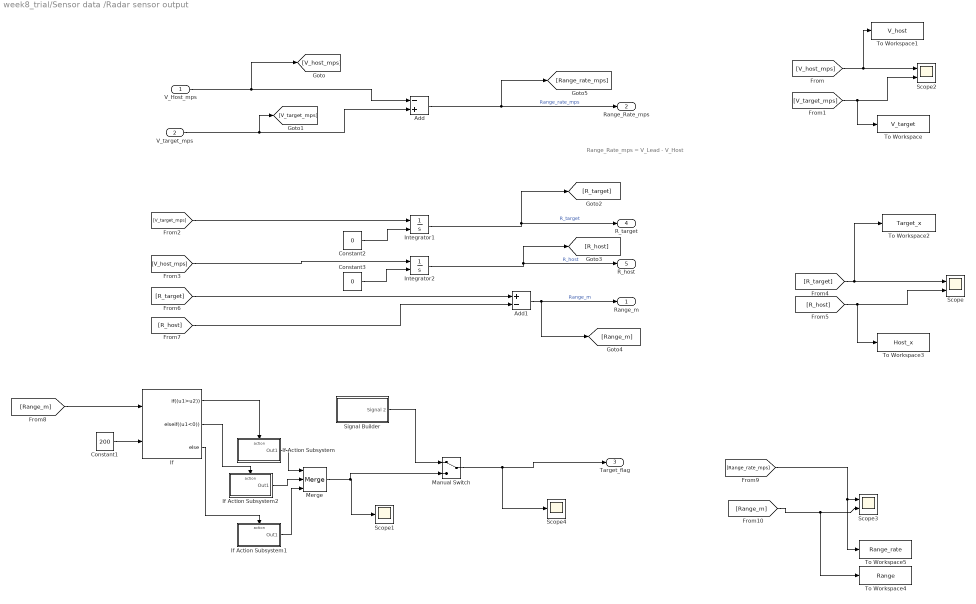
== system week8_trial/Sensor data /Radar sensor output ==
  note: Range_Rate_mps = V_Lead - V_Host
  V_Host_mps : Inport
  V_target_mps : Inport  Port=2
  Add : Sum  Inputs=-+
  Add1 : Sum  Inputs=+-
  Constant1 : Constant  Value=200
  Constant2 : Constant  Value=0
  Constant3 : Constant  Value=0
  If : If  NumInputs=2  IfExpression=(u1>u2)  ElseIfExpressions=(u1<0)
  If Action Subsystem : Subsystem  TreatAsAtomicUnit=on
  If Action Subsystem1 : Subsystem  TreatAsAtomicUnit=on
  If Action Subsystem2 : Subsystem  TreatAsAtomicUnit=on
  Integrator1 : Integrator  InitialConditionSource=external  InitialCondition=500
  Integrator2 : Integrator  InitialConditionSource=external
  Manual Switch : ManualSwitch
  Merge : Merge  Inputs=3
  Scope : Scope  NumInputPorts=2
  Scope1 : Scope
  Scope2 : Scope  NumInputPorts=2
  Scope3 : Scope  NumInputPorts=2
  Scope4 : Scope
  Signal Builder : Subsystem  Tag=STV Subsys  LoadFcn=sigbuilder_block('load');  StartFcn=sigbuilder_block('start');  StopFcn=sigbuilder_block('stop');  ClipboardFcn=sigbuilder_block('clipboard');  mask(Sigbuilder block){tuvar=[0:10]}
      mask help: Simulink:masks:SigbuilderBlock_MD
      mask init:
      | if ~strcmp(get_param(bdroot(gcbh),'SimulationStatus'),'stopped') tuvar = sigbuilder_block('maskInit'); end
      settings: CopyFcn=sigbuilder_block('copy');  DeleteFcn=sigbuilder_block('delete');  ModelCloseFcn=sigbuilder_block('modelClose');  PreSaveFcn=sigbuilder_block('preSave');  PauseFcn=sigbuilder_block('pause');  ContinueFcn=sigbuilder_block('continue');  NameChangeFcn=sigbuilder_block('namechange');  OpenFcn=sigbuilder_block('open',[1876.5 144 550.5 417.75 ]);  CloseFcn=sigbuilder_block('close');
      mask Display: plot(0, 0, 100, 100,[2, 2, 32, 32, 2], [68, 8, 8, 68, 68],[32, 2], [38, 38], [32, 19, 2],[53, 60, 44], [32, 17, 17, 2],[16, 16, 31, 31]);txt = getActiveGroup(gcbh);text(2, 100, txt,'verticalAlignment', 'top');
  To Workspace : ToWorkspace  VariableName=V_target  SampleTime=-1
  To Workspace1 : ToWorkspace  VariableName=V_host  SampleTime=-1
  To Workspace2 : ToWorkspace  VariableName=Target_x  SampleTime=-1
  To Workspace3 : ToWorkspace  VariableName=Host_x  SampleTime=-1
  To Workspace4 : ToWorkspace  VariableName=Range  SampleTime=-1
  To Workspace5 : ToWorkspace  VariableName=Range_rate  SampleTime=-1
  Range_m : Outport
  Range_Rate_mps : Outport  Port=2
  Target_flag : Outport  Port=3
  R_target : Outport  Port=4
  R_host : Outport  Port=5
  wires:
  V_target_mps/1 -> Add/2, [V_target_mps]
  V_Host_mps/1 -> Add/1, [V_host_mps]
  Add/1 -> [Range_rate_mps], Range_Rate_mps/1  "Range_rate_mps"
  Integrator1/1 -> [R_target], R_target/1  "R_target"
  Integrator2/1 -> [R_host], R_host/1  "R_host"
  Add1/1 -> [Range_m], Range_m/1  "Range_m"
  [V_host_mps] -> To Workspace1/1, Scope2/1
  [V_target_mps] -> To Workspace/1, Scope2/2
  [V_target_mps] -> Integrator1/1
  [V_host_mps] -> Integrator2/1
  [R_target] -> To Workspace2/1, Scope/1
  [R_host] -> To Workspace3/1, Scope/2
  [R_target] -> Add1/1
  [R_host] -> Add1/2
  [Range_rate_mps] -> To Workspace5/1, Scope3/1
  [Range_m] -> To Workspace4/1, Scope3/2
  Constant2/1 -> Integrator1/2
  Constant3/1 -> Integrator2/2
  If Action Subsystem/1(Out1) -> Merge/1
  If/1 -> If Action Subsystem/Action
  If Action Subsystem1/1(Out1) -> Merge/3
  Constant1/1 -> If/2
  If/3 -> If Action Subsystem1/Action
  [Range_m] -> If/1
  If/2 -> If Action Subsystem2/Action
  Merge/1 -> Manual Switch/2, Scope1/1
  If Action Subsystem2/1(Out1) -> Merge/2
  Manual Switch/1 -> Scope4/1, Target_flag/1
  Signal Builder/1(Signal 2) -> Manual Switch/1

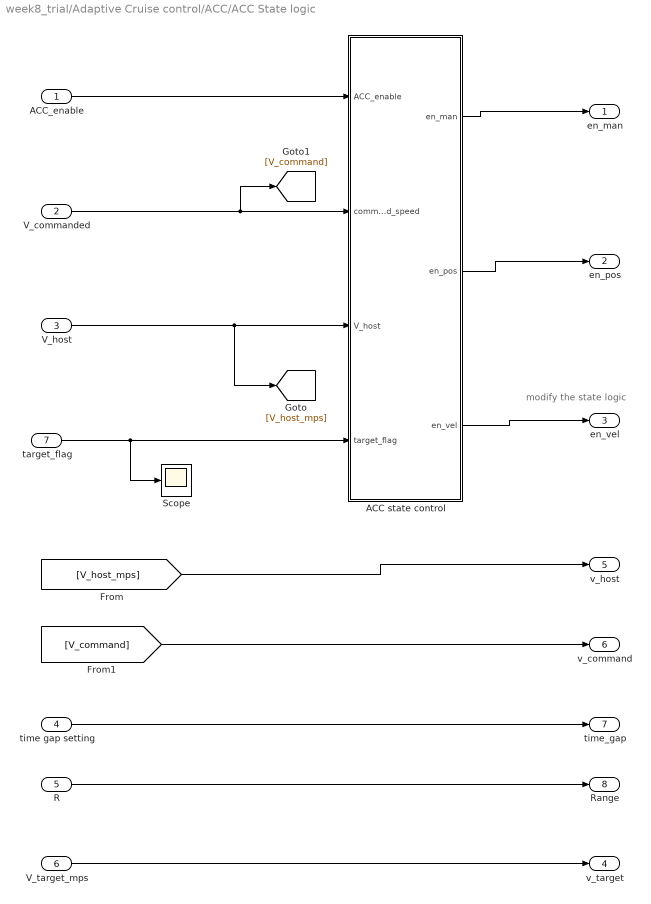
== system week8_trial/Adaptive Cruise control/ACC/ACC State logic ==
  note: modify the state logic
  ACC_enable : Inport
  V_commanded : Inport  Port=2
  V_host : Inport  Port=3
  time gap setting : Inport  Port=4
  R : Inport  Port=5
  V_target_mps : Inport  Port=6
  target_flag : Inport  Port=7
  ACC state control : Stateflow chart  TreatAsAtomicUnit=on
  Scope : Scope
  en_man : Outport
  en_pos : Outport  Port=2
  en_vel : Outport  Port=3
  v_target : Outport  Port=4
  v_host : Outport  Port=5
  v_command : Outport  Port=6
  time_gap : Outport  Port=7
  Range : Outport  Port=8
  wires:
  ACC state control/1(en_man) -> en_man/1
  ACC state control/2(en_pos) -> en_pos/1
  ACC state control/3(en_vel) -> en_vel/1
  ACC_enable/1 -> ACC state control/1(ACC_enable)
  V_commanded/1 -> [V_command], ACC state control/2(commanded_speed)
  V_target_mps/1 -> v_target/1
  V_host/1 -> [V_host_mps], ACC state control/3(V_host)
  target_flag/1 -> Scope/1, ACC state control/4(target_flag)
  [V_host_mps] -> v_host/1
  [V_command] -> v_command/1
  time gap setting/1 -> time_gap/1
  R/1 -> Range/1

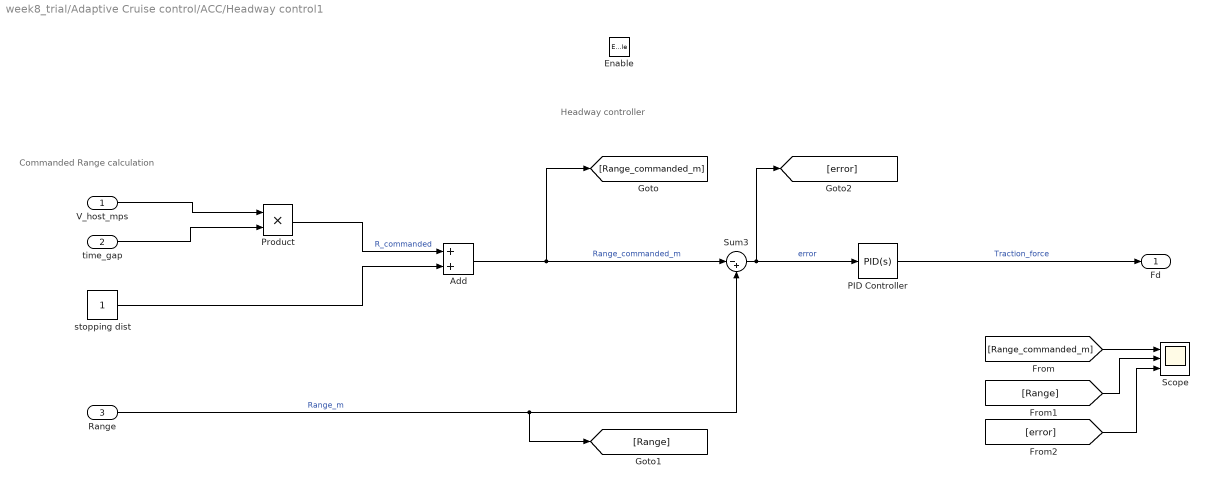
== system week8_trial/Adaptive Cruise control/ACC/Headway control1 ==
  note: Commanded Range calculation
  note: Headway controller
  V_host_mps : Inport
  time_gap : Inport  Port=2
  Range : Inport  Port=3
  Enable : EnablePort
  Add : Sum
  PID Controller : pid_lib/PID Controller  Controller=PID  Form=Parallel  TimeDomain=Continuous-time  UseExternalTs=off  SampleTime=-1  IntegratorMethod=Forward Euler  FilterMethod=Forward Euler  ControllerParametersSource=internal  P=100  I=3  D=950  UseFilter=on  N=75  TunerSelectOption=Transfer Function Based (PID Tuner App)  InitialConditionSource=internal  InitialConditionForIntegrator=0  InitialConditionForFilter=0  DifferentiatorICPrevScaledInput=0  ExternalReset=none  TrackingMode=off  Kt=1  LimitOutput=off  SatLimitsSource=internal  UpperSaturationLimit=inf  LowerSaturationLimit=-inf  LinearizeAsGain=on  AntiWindupMode=none  Kb=1  POutMin=[]  POutMax=[]  IOutMin=[]  IOutMax=[]  DOutMin=[]  DOutMax=[]  NOutMin=[]  NOutMax=[]  SumOutMin=[]  SumOutMax=[]  SaturationOutMin=[]  SaturationOutMax=[]  PParamMin=[]  PParamMax=[]  IParamMin=[]  IParamMax=[]  DParamMin=[]  DParamMax=[]  NParamMin=[]  NParamMax=[]  KbParamMin=[]  KbParamMax=[]  KtParamMin=[]  KtParamMax=[]  KbOutMin=[]  KbOutMax=[]  KtOutMin=[]  KtOutMax=[]  IntegratorOutMin=[]  IntegratorOutMax=[]  FilterOutMin=[]  FilterOutMax=[]  SumI1OutMin=[]  SumI1OutMax=[]  SumI2OutMin=[]  SumI2OutMax=[]  SumI3OutMin=[]  SumI3OutMax=[]  SumI4OutMin=[]  SumI4OutMax=[]  SumDOutMin=[]  SumDOutMax=[]  DifferentiatorOutMin=[]  DifferentiatorOutMax=[]  FilterDiffOutCoefMin=[]  FilterDiffOutCoefMax=[]  ReciprocalOutMin=[]  ReciprocalOutMax=[]  SumDenOutMin=[]  SumDenOutMax=[]  SumNumOutMin=[]  SumNumOutMax=[]  DivideOutMin=[]  DivideOutMax=[]  UdiffTsProdOutMin=[]  UdiffTsProdOutMax=[]  NTsProdOutMin=[]  NTsProdOutMax=[]  UintegralTsProdOutMin=[]  UintegralTsProdOutMax=[]  UngainTsProdOutMin=[]  UngainTsProdOutMax=[]  IntegratorContinuousStateAttributes=''  IntegratorStateMustResolveToSignalObject=off  IntegratorRTWStateStorageClass=Auto  FilterContinuousStateAttributes=''  FilterStateMustResolveToSignalObject=off  FilterRTWStateStorageClass=Auto  ParallelPVariant=InternalParameters  IdealPVariant=Disabled  IVariant=InternalParameters  DVariant=InternalParameters  IntegratorVariant=Continuous  SatVariant=Disabled  AWVariant=Passthrough  PCopyVariant=Disabled  TRVariant=Disabled  FdbkBlocksVariant=Forward  IdealPFdbkVariant=Disabled  SatFdbkVariant=Disabled  DerivativeFilterVariant=ContFilter  NVariant=InternalParameters  NCopyVariant=Disabled  FilterICVariant=InternalICsFilter  IntegratorICVariant=InternalICs  ExternalResetVariant=Disabled  TRSumVariant=Passthrough  SumFdbkVariant=Disabled  SumVariant=Sum_PID  TsampFilterVariant=InternalTs  TsampNgainVariant=Passthrough  TsampIntegralVariant=Passthrough  ExternalSaturationOutDataTypeStr=Inherit: Same as second input
  Product : Product
  Scope : Scope  NumInputPorts=3
  Sum3 : Sum  Inputs=|-+
  stopping dist : Constant
  Fd : Outport
  wires:
  stopping dist/1 -> Add/2
  PID Controller/1 -> Fd/1  "Traction_force"
  Product/1 -> Add/1  "R_commanded"
  time_gap/1 -> Product/2
  Add/1 -> [Range_commanded_m], Sum3/1  "Range_commanded_m"
  Range/1 -> [Range], Sum3/2  "Range_m"
  [Range] -> Scope/2
  [Range_commanded_m] -> Scope/1
  Sum3/1 -> [error], PID Controller/1  "error"
  [error] -> Scope/3
  V_host_mps/1 -> Product/1

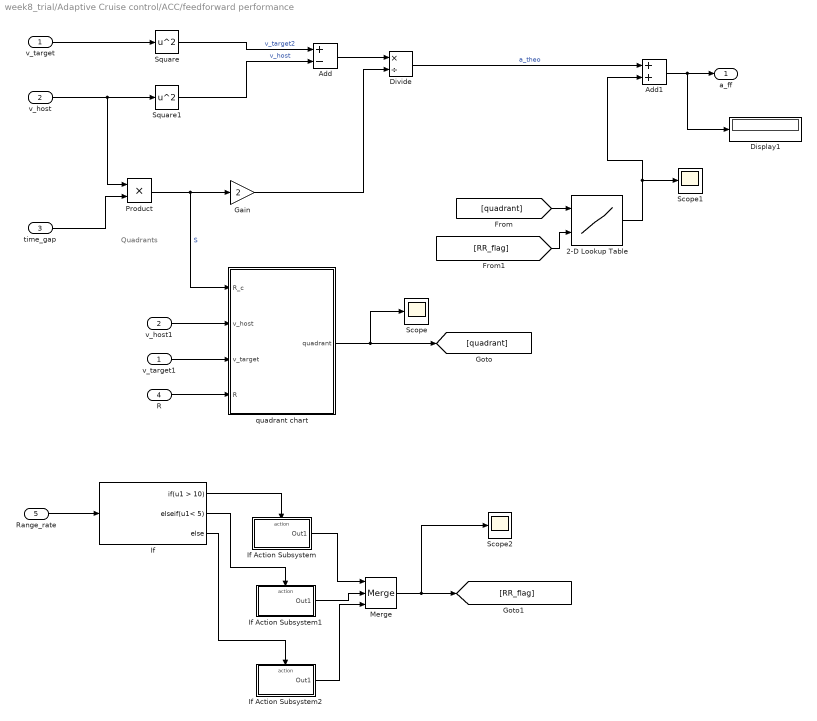
== system week8_trial/Adaptive Cruise control/ACC/feedforward performance ==
  note: Quadrants
  v_target : Inport
  v_host : Inport  Port=2
  time_gap : Inport  Port=3
  R : Inport  Port=4
  Range_rate : Inport  Port=5
  2-D Lookup Table : Lookup_n-D  BreakpointsForDimension1=[1,2,3,4]  BreakpointsForDimension2=[1,2,3]  Table=reshape([10,15,10,20,30,19,18,38,50,20,23,43],4,3)  InternalRulePriority=Speed  RndMeth=Simplest  InputSameDT=on
      settings: InputPortMap=u0,u1
  Add : Sum  Inputs=+-
  Add1 : Sum
  Display1 : Display
  Divide : Product  Inputs=*/
  Gain : Gain  Gain=2
  If : If  IfExpression=u1 > 10  ElseIfExpressions=u1< 5
  If Action Subsystem : Subsystem  TreatAsAtomicUnit=on
  If Action Subsystem1 : Subsystem  TreatAsAtomicUnit=on
  If Action Subsystem2 : Subsystem  TreatAsAtomicUnit=on
  Merge : Merge  Inputs=3
  Product : Product
  Scope : Scope
  Scope1 : Scope
  Scope2 : Scope
  Square : Math  Operator=square  SaturateOnIntegerOverflow=on
  Square1 : Math  Operator=square  SaturateOnIntegerOverflow=on
  quadrant chart : Stateflow chart  TreatAsAtomicUnit=on
  v_host1 : InportShadow  Port=2
  v_target1 : InportShadow
  a_ff : Outport
  wires:
  v_target/1 -> Square/1
  Square/1 -> Add/1  "v_target2"
  Square1/1 -> Add/2  "v_host"
  Add/1 -> Divide/1
  time_gap/1 -> Product/2
  Product/1 -> quadrant chart/1(R_c), Gain/1  "S"
  Gain/1 -> Divide/2
  v_host1/1 -> quadrant chart/2(v_host)
  v_target1/1 -> quadrant chart/3(v_target)
  R/1 -> quadrant chart/4(R)
  quadrant chart/1(quadrant) -> Scope/1, [quadrant]
  [quadrant] -> 2-D Lookup Table/1
  Add1/1 -> Display1/1, a_ff/1
  2-D Lookup Table/1 -> Scope1/1, Add1/2
  Divide/1 -> Add1/1  "a_theo"
  v_host/1 -> Product/1, Square1/1
  Range_rate/1 -> If/1
  [RR_flag] -> 2-D Lookup Table/2
  Merge/1 -> Scope2/1, [RR_flag]
  If/1 -> If Action Subsystem/Action
  If/2 -> If Action Subsystem1/Action
  If/3 -> If Action Subsystem2/Action
  If Action Subsystem/1(Out1) -> Merge/1
  If Action Subsystem1/1(Out1) -> Merge/2
  If Action Subsystem2/1(Out1) -> Merge/3

== system week8_trial/Adaptive Cruise control/ACC/manual control ==
  Input : Inport
  Enable : EnablePort
  Out1 : Outport
  wires:
  Input/1 -> Out1/1

== system week8_trial/Adaptive Cruise control/ACC/velocity control ==
  V_command : Inport
  V_host : Inport  Port=2
  Enable : EnablePort
  Add1 : Sum  Inputs=|+-
  PID controller : pid_lib/PID Controller  Controller=PID  Form=Parallel  TimeDomain=Continuous-time  UseExternalTs=off  SampleTime=-1  IntegratorMethod=Forward Euler  FilterMethod=Forward Euler  ControllerParametersSource=internal  P=350  I=8.132  D=0  UseFilter=on  N=75  TunerSelectOption=Transfer Function Based (PID Tuner App)  InitialConditionSource=internal  InitialConditionForIntegrator=0  InitialConditionForFilter=0  DifferentiatorICPrevScaledInput=0  ExternalReset=none  TrackingMode=off  Kt=1  LimitOutput=off  SatLimitsSource=internal  UpperSaturationLimit=inf  LowerSaturationLimit=-inf  LinearizeAsGain=on  AntiWindupMode=none  Kb=1  POutMin=[]  POutMax=[]  IOutMin=[]  IOutMax=[]  DOutMin=[]  DOutMax=[]  NOutMin=[]  NOutMax=[]  SumOutMin=[]  SumOutMax=[]  SaturationOutMin=[]  SaturationOutMax=[]  PParamMin=[]  PParamMax=[]  IParamMin=[]  IParamMax=[]  DParamMin=[]  DParamMax=[]  NParamMin=[]  NParamMax=[]  KbParamMin=[]  KbParamMax=[]  KtParamMin=[]  KtParamMax=[]  KbOutMin=[]  KbOutMax=[]  KtOutMin=[]  KtOutMax=[]  IntegratorOutMin=[]  IntegratorOutMax=[]  FilterOutMin=[]  FilterOutMax=[]  SumI1OutMin=[]  SumI1OutMax=[]  SumI2OutMin=[]  SumI2OutMax=[]  SumI3OutMin=[]  SumI3OutMax=[]  SumI4OutMin=[]  SumI4OutMax=[]  SumDOutMin=[]  SumDOutMax=[]  DifferentiatorOutMin=[]  DifferentiatorOutMax=[]  FilterDiffOutCoefMin=[]  FilterDiffOutCoefMax=[]  ReciprocalOutMin=[]  ReciprocalOutMax=[]  SumDenOutMin=[]  SumDenOutMax=[]  SumNumOutMin=[]  SumNumOutMax=[]  DivideOutMin=[]  DivideOutMax=[]  UdiffTsProdOutMin=[]  UdiffTsProdOutMax=[]  NTsProdOutMin=[]  NTsProdOutMax=[]  UintegralTsProdOutMin=[]  UintegralTsProdOutMax=[]  UngainTsProdOutMin=[]  UngainTsProdOutMax=[]  IntegratorContinuousStateAttributes=''  IntegratorStateMustResolveToSignalObject=off  IntegratorRTWStateStorageClass=Auto  FilterContinuousStateAttributes=''  FilterStateMustResolveToSignalObject=off  FilterRTWStateStorageClass=Auto  ParallelPVariant=InternalParameters  IdealPVariant=Disabled  IVariant=InternalParameters  DVariant=InternalParameters  IntegratorVariant=Continuous  SatVariant=Disabled  AWVariant=Passthrough  PCopyVariant=Disabled  TRVariant=Disabled  FdbkBlocksVariant=Forward  IdealPFdbkVariant=Disabled  SatFdbkVariant=Disabled  DerivativeFilterVariant=ContFilter  NVariant=InternalParameters  NCopyVariant=Disabled  FilterICVariant=InternalICsFilter  IntegratorICVariant=InternalICs  ExternalResetVariant=Disabled  TRSumVariant=Passthrough  SumFdbkVariant=Disabled  SumVariant=Sum_PID  TsampFilterVariant=InternalTs  TsampNgainVariant=Passthrough  TsampIntegralVariant=Passthrough  ExternalSaturationOutDataTypeStr=Inherit: Same as second input
  Scope : Scope  NumInputPorts=2
  Fd : Outport
  wires:
  Add1/1 -> PID controller/1
  V_command/1 -> Scope/1, Add1/1
  PID controller/1 -> Fd/1
  V_host/1 -> Scope/2, Add1/2

== system week8_trial/Adaptive Cruise control/LCA/MPC ==
  note: LATERAL CONTROL WITH MPC
  seq_curvature : Inport
  V_host_mps : Inport  Port=2
  lateral_deviation : Inport  Port=3
  relative_yaw_angle : Inport  Port=4
  Enable : EnablePort
  Lane Keeping Assist System : mpcadaslib/Lane Keeping Assist System  ModelType=Use vehicle parameters  VehicleMass=1140  VehicleYawInertia=1436.24  LengthToFront=1.165  LengthToRear=1.165  FrontTireStiffness=155494.663  RearTireStiffness=1554494.663  EgoModelMatrixA=[-4.4021 ,-12.4603;1.3913,-5.1868]  EgoModelMatrixB=[24.1270;15.8609]  EgoModelMatrixC=[1,0;0,1]  InitialLongVel=V_init  TransportLag=0  MinSteering=-0.5  umin_ext=off  MaxSteering=0.5  umax_ext=off  Ts=0.1  PredictionHorizon=10  ControllerBehavior=0.240  suboptimal=off  maxiter=10  datatypeopt=double  optmode=off  trackmode=off
      settings: SourceProductBaseCode=MP
  Scope : Scope
  Scope1 : Scope  NumInputPorts=3
  To Workspace : ToWorkspace  VariableName=cross_track  SampleTime=-1
  To Workspace1 : ToWorkspace  VariableName=Theta_e  SampleTime=-1
  steering angle (rad) : Outport
  wires:
  Lane Keeping Assist System/1 -> Scope/1, steering angle (rad)/1
  seq_curvature/1 -> Lane Keeping Assist System/1
  V_host_mps/1 -> Scope1/3, Lane Keeping Assist System/2
  lateral_deviation/1 -> Scope1/1, To Workspace/1, Lane Keeping Assist System/3
  relative_yaw_angle/1 -> Scope1/2, To Workspace1/1, Lane Keeping Assist System/4

== system week8_trial/Adaptive Cruise control/LCA/manual ==
  Enable : EnablePort
  Constant : Constant  Value=0
  delta : Outport
  wires:
  Constant/1 -> delta/1

== system week8_trial/Sensor data /Lateral control sensor inputs/Sensor Dynamics ==
  Current curvature : Inport
  Longitudinal velocity : Inport  Port=2
  Lateral velocity : Inport  Port=3
  Yaw rate : Inport  Port=4
  Integrator : Integrator
  Integrator2 : Integrator
  Mux1 : Mux  Inputs=[1 1 1]
  Product : Product
  Subtract : Sum  Inputs=-+
  e1dot : Fcn  Expr=u(1)*u(3)+u(2)
  Lateral deviation : Outport  VectorParamsAs1DForOutWhenUnconnected=off
  Relative yaw angle : Outport  Port=2  VectorParamsAs1DForOutWhenUnconnected=off
  wires:
  Current curvature/1 -> Product/2
  Integrator2/1 -> Mux1/3, Relative yaw angle/1  "e2"
  Mux1/1 -> e1dot/1
  e1dot/1 -> Integrator/1
  Longitudinal velocity/1 -> Product/1, Mux1/1
  Lateral velocity/1 -> Mux1/2
  Integrator/1 -> Lateral deviation/1  "e1"
  Product/1 -> Subtract/1
  Yaw rate/1 -> Subtract/2
  Subtract/1 -> Integrator2/1  "e2dot"

== system week8_trial/Sensor data /Lateral control sensor inputs/Subsystem ==
  MATLAB Function : MATLAB Function  TreatAsAtomicUnit=on
  Memory1 : Memory  InheritSampleTime=on  LinearizeAsDelay=on
  sequence : Outport  VectorParamsAs1DForOutWhenUnconnected=off
  current : Outport  Port=2  VectorParamsAs1DForOutWhenUnconnected=off
  wires:
  MATLAB Function/2(first) -> current/1
  MATLAB Function/3(next_t) -> Memory1/1
  MATLAB Function/1(seq) -> sequence/1
  Memory1/1 -> MATLAB Function/1(t)

== system week8_trial/Sensor data /Radar sensor output/If Action Subsystem ==
  Action Port : ActionPort  ActionPortLabel=if((u1>u2))
  Constant : Constant  Value=0
  Out1 : Outport
  wires:
  Constant/1 -> Out1/1

== system week8_trial/Sensor data /Radar sensor output/If Action Subsystem1 ==
  Action Port : ActionPort  ActionPortLabel=else
  Constant : Constant
  Out1 : Outport
  wires:
  Constant/1 -> Out1/1

== system week8_trial/Sensor data /Radar sensor output/If Action Subsystem2 ==
  Action Port : ActionPort  ActionPortLabel=elseif((u1<0))
  Constant : Constant  Value=0
  Out1 : Outport
  wires:
  Constant/1 -> Out1/1

== system week8_trial/Sensor data /Radar sensor output/Signal Builder ==
  Demux : Demux  Tag=STV Demux  Outputs=1
      settings: DisplayOption=none
  FromWs : FromWorkspace  Tag=STV FromWs  VariableName=tuvar
      SigBuilderData=|
      | common.afterFinalStr = 'Extrapolate'
      | common.sampleTime = 0
      | dataSet.timeRange = [0 100]
      | dataSet.name = 'Group 1'
      | sbobj.Groups.Name = 'Group 1'
      | sbobj.Groups.Signals.Name = 'Signal 2'
      | sbobj.Groups.Signals.XData = [0 29.8 29.8 100]
      | sbobj.Groups.Signals.YData = [0 0 1 1]
      | sbobj.Groups.TimeRange = [0 100]
  Signal 2 : Outport  Tag=STV Outport
  wires:
  FromWs/1 -> Demux/1
  Demux/1 -> Signal 2/1

== system week8_trial/Adaptive Cruise control/ACC/feedforward performance/If Action Subsystem ==
  Action Port : ActionPort  ActionPortLabel=if(u1 > 10)
  Constant : Constant
  Out1 : Outport
  wires:
  Constant/1 -> Out1/1

== system week8_trial/Adaptive Cruise control/ACC/feedforward performance/If Action Subsystem1 ==
  Action Port : ActionPort  ActionPortLabel=elseif(u1< 5)
  Constant : Constant  Value=3
  Out1 : Outport
  wires:
  Constant/1 -> Out1/1

== system week8_trial/Adaptive Cruise control/ACC/feedforward performance/If Action Subsystem2 ==
  Action Port : ActionPort  ActionPortLabel=else
  Constant : Constant  Value=2
  Out1 : Outport
  wires:
  Constant/1 -> Out1/1
